simulink model "alpha_closed"  (R2021b)
settings: Solver=VariableStepAuto  StartTime=0.0  StopTime=TF  RelTol=1e-3
values from neighbouring files (symbols this model uses):
  deltaA = 0    [RunAircraftStabilityAxesModel.m]
  deltaE = -0.1    [RunAircraftStabilityAxesModel.m]
  deltaR = 0    [RunAircraftStabilityAxesModel.m]
  deltaT1 = 0.08    [RunAircraftStabilityAxesModel.m]
  deltaT2 = 0.08    [RunAircraftStabilityAxesModel.m]
  X0 = [VT0; alpha0; theta0; Q0;beta0 ;phi0 ; P0; R0; psi0]    [RunAircraftStabilityAxesModel.m]
undefined symbols (not defined in the file or in its folder): StabilityAxesModel
settings Model: Creator=mo112  LastModifiedBy=mo112

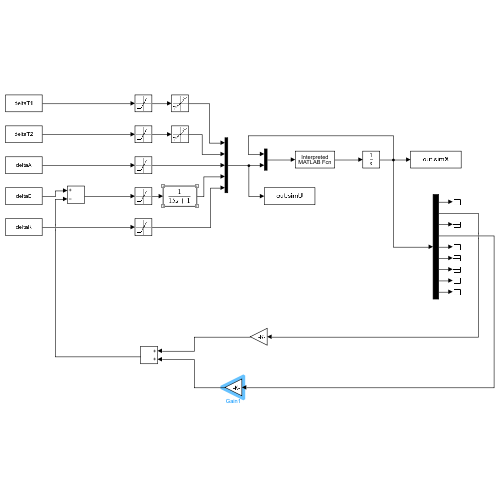
[thumbnail: Simulink's stored preview of the top-level diagram]
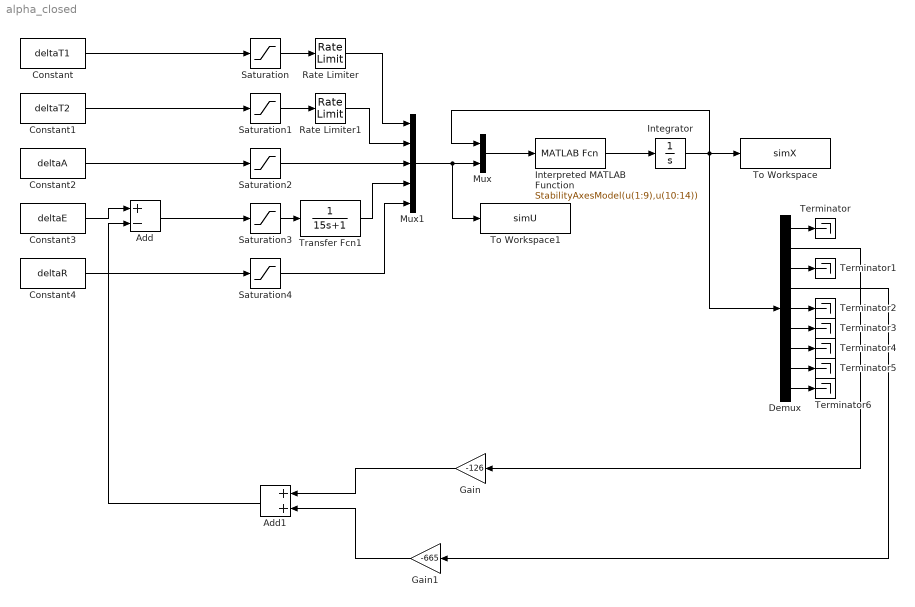
== system alpha_closed ==
  Add : Sum  Inputs=+-
  Add1 : Sum
  Constant : Constant  Value=deltaT1
  Constant1 : Constant  Value=deltaT2
  Constant2 : Constant  Value=deltaA
  Constant3 : Constant  Value=deltaE
  Constant4 : Constant  Value=deltaR
  Demux : Demux  Outputs=9
  Gain : Gain  Gain=-126
  Gain1 : Gain  Gain=-665
  Integrator : Integrator  InitialCondition=X0
  Interpreted MATLAB Function : MATLABFcn  MATLABFcn=StabilityAxesModel(u(1:9),u(10:14))
  Mux : Mux  Inputs=2
  Mux1 : Mux  Inputs=5
  Rate Limiter : RateLimiter  RisingSlewLimit=1.6  FallingSlewLimit=-1.6  SampleTimeMode=inherited
  Rate Limiter1 : RateLimiter  RisingSlewLimit=1.6  FallingSlewLimit=-1.6  SampleTimeMode=inherited
  Saturation : Saturate  UpperLimit=1*(pi/180)  LowerLimit=0.5*(pi/180)
  Saturation1 : Saturate  UpperLimit=1*(pi/180)  LowerLimit=0.5*(pi/180)
  Saturation2 : Saturate  UpperLimit=25*(pi/180)  LowerLimit=-25*(pi/180)
  Saturation3 : Saturate  UpperLimit=10*(pi/180)  LowerLimit=-25*(pi/180)
  Saturation4 : Saturate  UpperLimit=30*(pi/180)  LowerLimit=-30*(pi/180)
  Terminator{,1..6} (7 alike) : Terminator
  To Workspace : ToWorkspace  VariableName=simX  SaveFormat=Timeseries  SampleTime=-1
  To Workspace1 : ToWorkspace  VariableName=simU  SaveFormat=Timeseries  SampleTime=-1
  Transfer Fcn1 : TransferFcn  Denominator=[15 1]
  wires:
  Integrator/1 -> Demux/1, To Workspace/1, Mux/1
  Mux1/1 -> To Workspace1/1, Mux/2
  Saturation1/1 -> Rate Limiter1/1
  Mux/1 -> Interpreted MATLAB Function/1
  Saturation2/1 -> Mux1/3
  Rate Limiter1/1 -> Mux1/2
  Constant/1 -> Saturation/1
  Saturation/1 -> Rate Limiter/1
  Rate Limiter/1 -> Mux1/1
  Constant2/1 -> Saturation2/1
  Constant4/1 -> Saturation4/1
  Interpreted MATLAB Function/1 -> Integrator/1
  Saturation4/1 -> Mux1/5
  Constant1/1 -> Saturation1/1
  Constant3/1 -> Add/1
  Transfer Fcn1/1 -> Mux1/4
  Saturation3/1 -> Transfer Fcn1/1
  Add/1 -> Saturation3/1
  Demux/2 -> Gain/1
  Demux/4 -> Gain1/1
  Gain1/1 -> Add1/2
  Gain/1 -> Add1/1
  Add1/1 -> Add/2
  Demux/1 -> Terminator/1
  Demux/3 -> Terminator1/1
  Demux/5 -> Terminator2/1
  Demux/6 -> Terminator3/1
  Demux/7 -> Terminator4/1
  Demux/8 -> Terminator5/1
  Demux/9 -> Terminator6/1
